simulink model "tvcModel"  (R2024b)
settings: Solver=VariableStepAuto  StartTime=0.0  StopTime=8  RelTol=1e-3
undefined symbols (not defined in the file): mass, max_speed, measurement_delay, movement_delay
libraries: shared6dof x1
settings Model: Creator=Sebastian Bagley  LastModifiedBy=Sebastian Bagley

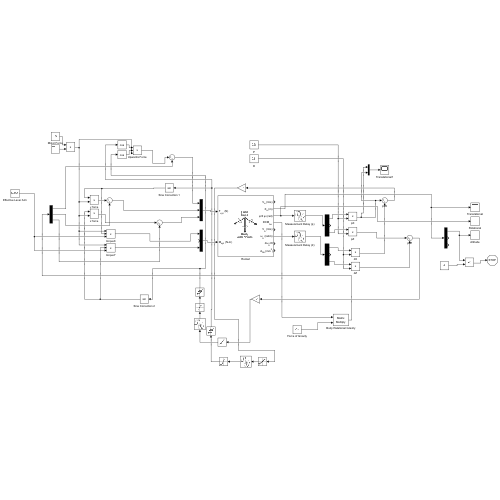
[thumbnail: Simulink's stored preview of the top-level diagram]
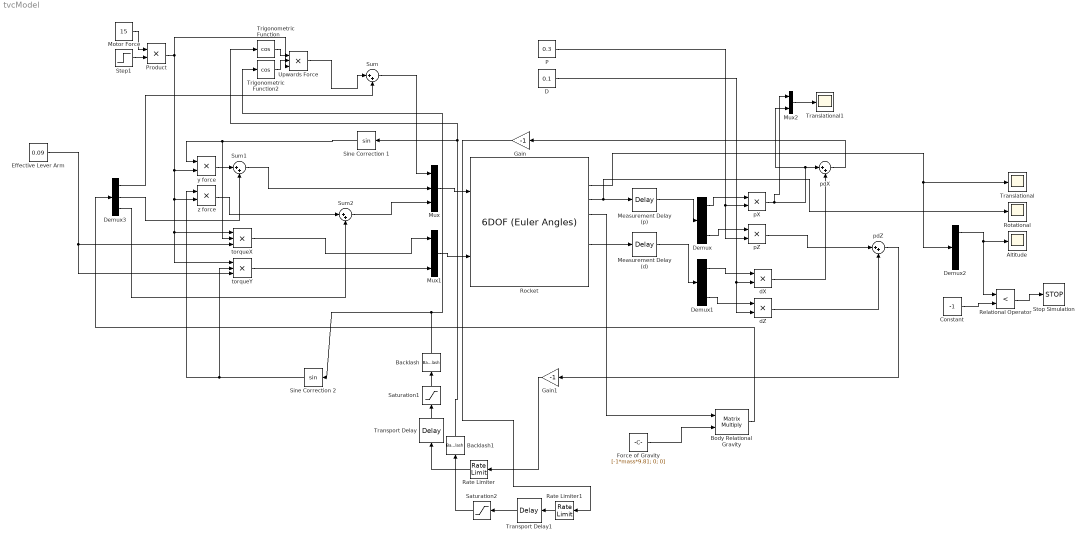
== system tvcModel ==
  Altitude : Scope
  Backlash : Backlash  BacklashWidth=backlash
  Backlash1 : Backlash  BacklashWidth=backlash
  Body Relational Gravity : Product  Multiplication=Matrix(*)
  Constant : Constant  Value=-1
  D : Constant  Value=0.1
  Demux{,1..3} (4 alike) : Demux  Outputs=3
  Effective Lever Arm : Constant  Value=0.09
  Force of Gravity : Constant  Value=[-1*mass*9.81; 0; 0]
  Gain : Gain  Gain=-1
  Gain1 : Gain  Gain=-1
  Measurement Delay (d) : TransportDelay  DelayTime=measurement_delay
  Measurement Delay (p) : TransportDelay  DelayTime=measurement_delay
  Motor Force : Constant  Value=15
  Mux : Mux  Inputs=3
  Mux1 : Mux  Inputs=3
  Mux2 : Mux  Inputs=2
  P : Constant  Value=0.3
  Product : Product
  Rate Limiter : RateLimiter  RisingSlewLimit=max_speed  FallingSlewLimit=-max_speed  SampleTimeMode=inherited
  Rate Limiter1 : RateLimiter  RisingSlewLimit=max_speed  FallingSlewLimit=-max_speed  SampleTimeMode=inherited
  Relational Operator : RelationalOperator  Operator=<  OutDataTypeStr=boolean  RndMeth=Simplest  InputSameDT=off
  Rocket : shared6dof/6DOF (Euler Angles)  units=Metric (MKS)  mtype=Fixed  rep=Euler Angles  xme_0=[0 0 0]  Vm_0=[0 0 0]  eul_0=[-0.5 0 0.5]  pm_0=[0 0 0]  mass_0=mass  mass_e=0.5  mass_f=2.0  inertia=[0.1, 0, 0; 0, 0.009719, 0; 0, 0, 0.1]  inertia_e=eye(3)  inertia_f=2*eye(3)  k_quat=1.0  vre_flag=on  abi_flag=off  aMode=0  xme_statename=''  Vm_statename=''  eul_statename=''  quat_statename=''  pm_statename=''  mass_statename=''
  Rotational : Scope
  Saturation1 : Saturate  UpperLimit=0.185  LowerLimit=-0.396
  Saturation2 : Saturate  UpperLimit=0.224  LowerLimit=-0.143
  Sine Correction 1 : Trigonometry
  Sine Correction 2 : Trigonometry
  Step1 : Step  Time=3.44  Before=1  After=0  SampleTime=0.01
  Stop Simulation : Stop
  Sum : Sum  Inputs=|++
  Sum1 : Sum  Inputs=|++
  Sum2 : Sum  Inputs=|++
  Translational : Scope
  Translational1 : Scope
  Transport Delay : TransportDelay  DelayTime=movement_delay
  Transport Delay1 : TransportDelay  DelayTime=movement_delay
  Trigonometric Function : Trigonometry  Operator=cos
  Trigonometric Function2 : Trigonometry  Operator=cos
  Upwards Force : Product  Inputs=3
  dX : Product
  dZ : Product
  pX : Product
  pZ : Product
  pdX : Sum  Inputs=|++
  pdZ : Sum  Inputs=|++
  torqueX : Product  Inputs=3
  torqueY : Product  Inputs=3
  y force : Product
  z force : Product
  wires:
  Motor Force/1 -> Product/1
  Mux/1 -> Rocket/1
  Step1/1 -> Product/2
  Rocket/2 -> Translational/1, Demux2/1
  Mux1/1 -> Rocket/2
  Rocket/3 -> Measurement Delay (p)/1, Rotational/1
  Demux/1 -> pX/1
  P/1 -> pZ/2, pX/2
  Demux/3 -> pZ/1
  Rocket/6 -> Measurement Delay (d)/1
  D/1 -> dZ/2, dX/2
  Demux1/1 -> dX/1
  Demux1/3 -> dZ/1
  torqueX/1 -> Mux1/1
  pdX/1 -> Gain/1
  Product/1 -> Upwards Force/3, torqueY/1, torqueX/1, z force/2, y force/2
  torqueY/1 -> Mux1/3
  pdZ/1 -> Gain1/1
  Gain/1 -> Rate Limiter1/1
  Gain1/1 -> Rate Limiter/1
  Sine Correction 2/1 -> z force/1, torqueY/2
  Sine Correction 1/1 -> torqueX/2, y force/1
  Trigonometric Function/1 -> Upwards Force/1
  Trigonometric Function2/1 -> Upwards Force/2
  Rocket/4 -> Body Relational Gravity/1
  Force of Gravity/1 -> Body Relational Gravity/2
  Body Relational Gravity/1 -> Demux3/1
  Upwards Force/1 -> Sum/1
  Sum/1 -> Mux/1
  Demux3/1 -> Sum/2
  y force/1 -> Sum1/1
  Sum1/1 -> Mux/2
  Demux3/2 -> Sum1/2
  z force/1 -> Sum2/1
  Sum2/1 -> Mux/3
  Demux3/3 -> Sum2/2
  Rate Limiter/1 -> Transport Delay/1
  Transport Delay/1 -> Saturation1/1
  Saturation1/1 -> Backlash/1
  Demux2/1 -> Relational Operator/1, Altitude/1
  Constant/1 -> Relational Operator/2
  Relational Operator/1 -> Stop Simulation/1
  Rate Limiter1/1 -> Transport Delay1/1
  Transport Delay1/1 -> Saturation2/1
  Effective Lever Arm/1 -> torqueX/3, torqueY/3
  Backlash/1 -> Trigonometric Function2/1, Sine Correction 2/1
  Backlash1/1 -> Trigonometric Function/1, Sine Correction 1/1
  Saturation2/1 -> Backlash1/1
  Measurement Delay (p)/1 -> Demux/1
  Measurement Delay (d)/1 -> Demux1/1
  dX/1 -> pdX/2
  dZ/1 -> pdZ/2
  pX/1 -> Mux2/2, pdX/1, Mux2/1
  pZ/1 -> pdZ/1
  Mux2/1 -> Translational1/1
